simulink model "e_131"  (R2018a)
settings: Solver=VariableStepAuto  StartTime=0.0  StopTime=ttotal  RelTol=1e-3
values from neighbouring files (symbols this model uses):
  b = 0    [e_11.m]    (also in e_12.m = 0.025; e_13.m; lab2.m)
  f = 0    [e_11.m]    (also in e_12.m = 1; e_13.m = 1; lab2.m = 1)
  k1 = 1/yl    [cont_10.m]    (also in e_10.m = 1/yl(n); e_11.m = 5; e_12.m = 5; e_13.m = 5)
  k2 = sqrt(2*k1)    [cont_10.m]    (also in e_10.m; e_11.m; e_12.m; e_13.m)
  yl = [0, 0.2, 0.4]    [e_10.m]    (also in e_11.m = 0.2; e_12.m = 0.2; e_13.m = 0.2; lab2.m = 0.2)
undefined symbols (not defined in the file or in its folder): sgn
settings Model: Creator=Carlos  LastModifiedBy=Carlos

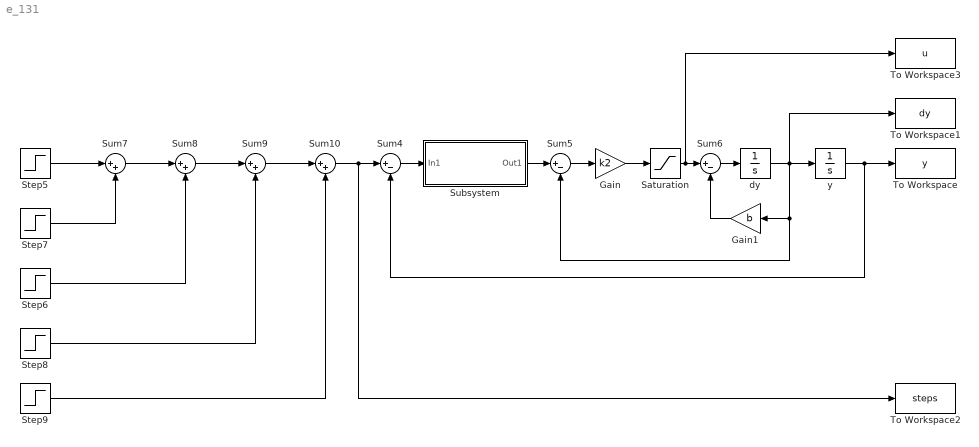
== system e_131 ==
  Gain : Gain  Gain=k2
  Gain1 : Gain  Gain=b
  Saturation : Saturate  UpperLimit=1  LowerLimit=-1
  Step5 : Step  SampleTime=0
  Step6 : Step  Time=10  After=2  SampleTime=0
  Step7 : Step  Time=6  After=-1  SampleTime=0
  Step8 : Step  Time=14  After=-1  SampleTime=0
  Step9 : Step  Time=18  SampleTime=0
  Subsystem : Subsystem
  Sum{7..10} (4 alike) : Sum  Inputs=|++
  Sum4 : Sum  Inputs=|+-
  Sum5 : Sum  Inputs=|+-
  Sum6 : Sum  Inputs=|+-
  To Workspace : ToWorkspace  VariableName=y  SampleTime=-1
  To Workspace1 : ToWorkspace  VariableName=dy  SampleTime=-1
  To Workspace2 : ToWorkspace  VariableName=steps  SampleTime=-1
  To Workspace3 : ToWorkspace  VariableName=u  SampleTime=-1
  dy : Integrator
  y : Integrator  InitialCondition=1
  wires:
  Gain1/1 -> Sum6/2
  y/1 -> Sum4/2, To Workspace/1
  Sum6/1 -> dy/1
  Saturation/1 -> To Workspace3/1, Sum6/1
  Gain/1 -> Saturation/1
  Sum4/1 -> Subsystem/1(In1)
  dy/1 -> To Workspace1/1, Gain1/1, Sum5/2, y/1
  Subsystem/1(Out1) -> Sum5/1
  Sum5/1 -> Gain/1
  Sum10/1 -> Sum4/1, To Workspace2/1
  Sum9/1 -> Sum10/1
  Step7/1 -> Sum7/2
  Step5/1 -> Sum7/1
  Sum8/1 -> Sum9/1
  Sum7/1 -> Sum8/1
  Step8/1 -> Sum9/2
  Step9/1 -> Sum10/2
  Step6/1 -> Sum8/2

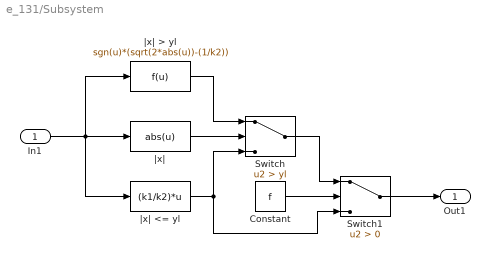
== system e_131/Subsystem ==
  In1 : Inport
  Constant : Constant  Value=f
  Switch : Switch  Criteria=u2 > Threshold  Threshold=yl
  Switch1 : Switch  Criteria=u2 > Threshold  ZeroCross=off
  |x| : Fcn  Expr=abs(u)
  |x| <= yl : Fcn  Expr=(k1/k2)*u
  |x| > yl : Fcn  Expr=sgn(u)*(sqrt(2*abs(u))-(1/k2))
  Out1 : Outport
  wires:
  In1/1 -> |x| <= yl/1, |x| > yl/1, |x|/1
  |x|/1 -> Switch/2
  |x| > yl/1 -> Switch/1
  |x| <= yl/1 -> Switch1/3, Switch/3
  Switch1/1 -> Out1/1
  Constant/1 -> Switch1/2
  Switch/1 -> Switch1/1
